simulink model "prius_rulebased"  (Simulink 9.0)
settings: Solver=ode4  StartTime=0.0  StopTime=time_final  FixedStep=time_step  RelTol=1e-3  AbsTol=1e-6
values from neighbouring files (symbols this model uses):
  A_frontal = 2.52    [prius_sim_data.m]
  C_d = 0.3    [prius_sim_data.m]
  enable_stop = 1    [prius_sim_data.m]
  eng_consum_fuel = [0 0.654 0.328 0.238 0.232 0.257 0.29 0.323 0.353 0.381 0.407 0.435 0.465 0.501 0.545 0.599 0.665 0.746 0.842 0.957 ... (first row only)    [prius_sim_data.m]
  eng_ctrl_max_trq = [77.33 78.2 79.07 79.94 80.81 81.68 82.35 82.85 83.35 83.85              84.35 84.83 85.2 85.58 85.95 86.32 86.7 87.13 87.6 88.08 88.55              89.02 89.47 89.79 90.11 90.43 90.76 91.08 91.4 91.73 92.05 92.38              92.7 93.03 93.35 93.67 93.99 94.32 94.64 94.96 95.29 95.61 95.93              96.26 96.58 96.9 97.22 97.55 97.87 98.19 98.52 98.84 99.17 99.49              99.81 100.2 100.5 ...(+23 chars)    [prius_sim_init.m]
  eng_idle_spd = 1000*pi/30    (= 104.71975512)    [prius_sim_init.m]
  eng_pwr_max = 40000    [prius_sim_init.m]
  eng_pwr_opt = eng_spd_opt.*eng_ctrl_max_trq*0.9    [prius_sim_init.m]
  eng_spd_opt = eng_ctrl_spd    [prius_sim_init.m]
  ess_cap_scale = 1    [prius_sim_data.m]
  ess_fixtemp = 40    [prius_sim_data.m]
  ess_init_soc = soc_init_index(simrun)    [prius_sim_init.m]
  ess_max_ah_cap = [6.0 6.0]    [prius_sim_data.m]
  ess_max_volts = 9    [prius_sim_data.m]
  ess_min_volts = 6    [prius_sim_data.m]
  ess_module_num = 40    [prius_sim_data.m]
  ess_res_scale_coef = [1 0 1 0]    [prius_sim_data.m]
  ess_res_scale_fun = inline('(x(1)*ess_module_num+x(2))/(x(3)*ess_cap_scale+x(4))','x','ess_module_num','ess_cap_scale')    [prius_sim_data.m]
  ess_tmp = [0 25]    [prius_sim_data.m]
  f_rolling = 0.015    [prius_sim_data.m]
  FR = 3.905    [prius_sim_data.m]
  g_eff_map = 0.95*[ 0.88	0.89	0.90	0.91	0.90	0.79	0.79	0.79	0.90	0.91	0.90	0.89	0.88 ... (first row only)    [prius_sim_data.m]
  g_gravity = 9.81    [prius_sim_data.m]
  g_max_spd = [-200000 -10000 -8000 -6500 -5500 -4000 -3500 -3000 -2500 -2000 -1500 -1000 -500 0 500 1000 1500 2000 2500 3000 3500 4000 5500 6500 8000 10000 200000]*(2*pi)/60    [prius_sim_data.m]
  g_max_trq = 1.2*[0.01 14.3 18 22 26 36 41 48 55 55 55 55 55 55 55 55 55 55 55 48 41 36 26 22 18 14.3 0.01]    [prius_sim_data.m]
  gc_ki_on = 0.005    [prius_sim_init.m]
  gc_kp_on = 0.9    [prius_sim_init.m]
  gear_no = 4    [prius_sim_data.m]
  Kp_c = 30    [prius_sim_init.m]
  m_eff_map = 0.95*[ .905    .905    .905    .905    .905    .905    .905    .905    .905    .905    .905    .905	.905    .905    .905    .905    .905    .905    .905    .905    .905    .905    .905 ... (first row only)    [prius_sim_data.m]
  m_map_spd = [0 500 1000 1500 2000 2500 3000 3500 4000 4500  6000]*(2*pi)/60    [prius_sim_data.m]
  m_max_trq = interp1(m_spd_data,m_max_trq_data,m_map_spd,'linear')    [prius_sim_data.m]
  m_min_volts = 60    [prius_sim_data.m]
  M_total = 1.254*10^3    (= 1254)    [prius_sim_data.m]
  max_gen_spd = 6500*pi/30    (= 680.678408278)    [prius_sim_init.m]
  min_gen_spd = -6500*pi/30    (= -680.678408278)    [prius_sim_init.m]
  P_eng_mode = 40000    [prius_sim_init.m]
  P_ev_mode = 12000    [prius_sim_init.m]
  R_tire = 0.287    [prius_sim_data.m]
  regstop_soc = 0.8    [prius_sim_init.m]
  rho_air = 1.2    [prius_sim_data.m]
  soc_control = 0.55    [prius_sim_init.m]
  T2W = inv(W2T)    [prius_sim_data.m]
  target_soc = 0.6    [prius_sim_init.m]
  Ti_c = 60    [prius_sim_init.m]
  time_final = 1*length(cyc_mph(:,2))-1    [prius_sim_init.m]
  Tt_c = 65    [prius_sim_init.m]
  tx_pg_r = 78    [prius_sim_data.m]
  tx_pg_s = 30    [prius_sim_data.m]
  v_max_c = 100    [prius_sim_init.m]
  w_engine_on = 30*1600/3600/R_tire    [prius_sim_init.m]
undefined symbols (not defined in the file or in its folder): eng_map_trq
undefined symbols (not defined in the file): ess_r_chg, ess_r_dis, ess_soc, ess_voc
(part 1 of 2)
settings Model: SuppressorTable=22 serialization::archive 11 0 6 0 0 0 0 0  Creator=Yifan  LastModifiedBy=Yifan  ExtModeTrigMode=oneshot  ExtModeArmWhenConnect=off
settings SolverCC: InitialStep=0.001
settings DataIOCC: SignalLoggingSaveFormat=ModelDataLogs  SaveOutput=off  SaveTime=off  SignalLoggingName=sigsOut
settings OptimizationCC: BooleanDataType=off  OptimizeBlockIOStorage=off  BufferReuse=off  GlobalBufferReuse=off  ExpressionFolding=off  LocalBlockOutputs=off  InitFltsAndDblsToZero=on
settings DebuggingCC: SaveWithParameterizedLinksMsg=none  SignalResolutionControl=TryResolveAllWithWarning  MultiTaskDSMMsg=warning  MultiTaskCondExecSysMsg=none
settings HardwareCC: TargetUnknown=on
settings GRTTargetCC: TargetFcnLib=ansi_tfl_tmw.mat  CombineOutputUpdateFcns=off  GRTInterface=on

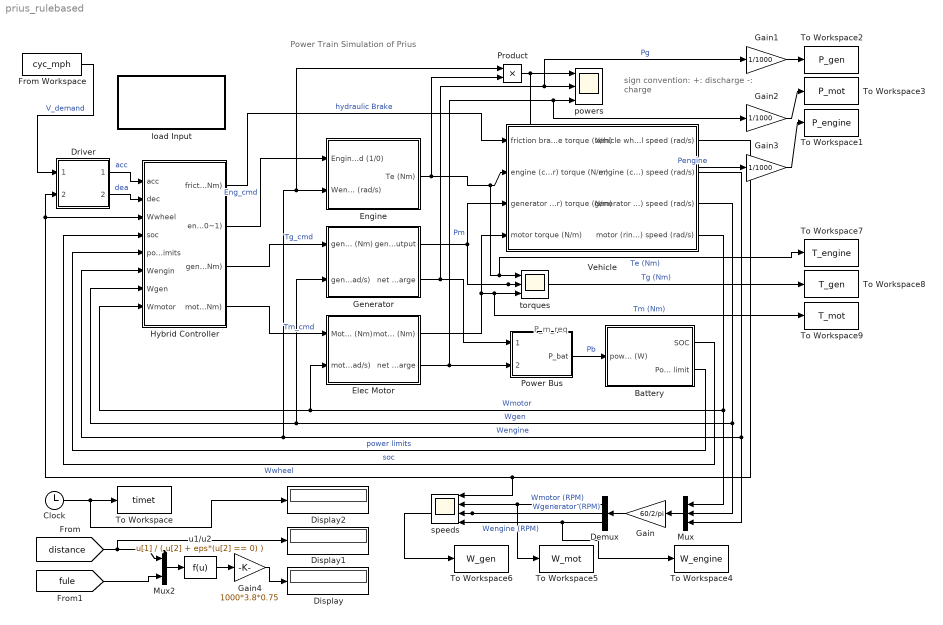
== system prius_rulebased ==
  note: Power Train Simulation of Prius
  note: P_m_req
  note: sign convention:
      | +: discharge     -: charge
  Battery : Subsystem
      mask Display: disp('Battery')
  Clock : Clock
  Demux : Demux  Outputs=3
  Display : Display
  Display1 : Display
  Display2 : Display
  "Driver " : Subsystem
      mask Display: disp('Driver')
  Elec Motor : Subsystem
      mask Display: disp('Electric\nMotor')
  Engine : Subsystem
      mask Display: disp('Engine')
  From Workspace : FromWorkspace  VariableName=cyc_mph  SampleTime=0
  Gain : Gain  Gain=60/2/pi  SaturateOnIntegerOverflow=on  OutDataTypeStr=Inherit: Same as input  ParamDataTypeStr=Inherit: Same as input
  Gain1 : Gain  Gain=1/1000  SaturateOnIntegerOverflow=on  OutDataTypeStr=Inherit: Same as input  ParamDataTypeStr=Inherit: Same as input
  Gain2 : Gain  Gain=1/1000  SaturateOnIntegerOverflow=on  OutDataTypeStr=Inherit: Same as input  ParamDataTypeStr=Inherit: Same as input
  Gain3 : Gain  Gain=1/1000  SaturateOnIntegerOverflow=on  OutDataTypeStr=Inherit: Same as input  ParamDataTypeStr=Inherit: Same as input
  Gain4 : Gain  Gain=1000*3.8*0.75  SaturateOnIntegerOverflow=on  OutDataTypeStr=Inherit: Same as input  ParamDataTypeStr=Inherit: Same as input
  Generator : Subsystem
      mask Display: disp('Generator')
  Hybrid Controller : Subsystem
      mask Display: disp('Hybrid\nController')
  Mux : Mux  Inputs=3
  Mux2 : Mux  Inputs=2
  Power Bus : Subsystem
      mask Display: disp('Power\nBus')
  Product : Product  SaturateOnIntegerOverflow=on  OutDataTypeStr=Inherit: Same as first input
  To Workspace : ToWorkspace  VariableName=timet  SampleTime=-1
  To Workspace1 : ToWorkspace  VariableName=P_engine  SampleTime=-1
  To Workspace2 : ToWorkspace  VariableName=P_gen  SampleTime=-1
  To Workspace3 : ToWorkspace  VariableName=P_mot  SampleTime=-1
  To Workspace4 : ToWorkspace  VariableName=W_engine  SampleTime=-1
  To Workspace5 : ToWorkspace  VariableName=W_mot  SampleTime=-1
  To Workspace6 : ToWorkspace  VariableName=W_gen  SampleTime=-1
  To Workspace7 : ToWorkspace  VariableName=T_engine  SampleTime=-1
  To Workspace8 : ToWorkspace  VariableName=T_gen  SampleTime=-1
  To Workspace9 : ToWorkspace  VariableName=T_mot  SampleTime=-1
  Vehicle : Subsystem
      mask Display: disp('Planetary Gear Set\n&\nVehicle')
  load Input : Subsystem
      settings: OpenFcn=prius_sim_init
      mask Help: This block runs/ndes_init.m file in the main directory
      mask Display: disp('Load Input Data')
  powers : Scope  NumInputPorts=3
  speeds : Scope  NumInputPorts=4
  torques : Scope  NumInputPorts=3
  u1/u2 : Fcn  Expr=u[1] / ( u[2] + eps*(u[2] == 0) )
  wires:
  Power Bus/1(P_bat) -> Battery/1(power req'd into bus (W))  "Pb"
  Battery/1(SOC) -> Hybrid Controller/4(soc)  "soc"
  Hybrid Controller/2(engine command (0~1)) -> Engine/1(Engine on/off cmd (1/0))  "Eng_cmd"
  Hybrid Controller/3(generator torque command (Nm)) -> Generator/1(generator command Torque (Nm))  "Tg_cmd"
  Hybrid Controller/4(motor torque command (Nm)) -> Elec Motor/1(Motor demand Torque (Nm))  "Tm_cmd"
  Elec Motor/2(net Power >0 discharge  <0 charge) -> Power Bus/2(P_motor), powers/3, Gain2/1  "Pm"
  Generator/2(net Power <0 discharge  >0 charge) -> Power Bus/1(P_generator), powers/2, Gain1/1  "Pg"
  Hybrid Controller/1(friction brake torque (Nm)) -> Vehicle/1(friction brake torque (N/m))  "hydraulic Brake"
  Engine/1(Te (Nm)) -> torques/1, To Workspace7/1, Vehicle/2(engine (carrier) torque (N/m)), Product/2  "Te (Nm)"
  Vehicle/1(vehicle wheel speed (rad/s)) -> speeds/1, "Driver "/2(Velocity (rad/s)), Hybrid Controller/3(Wwheel)  "Wwheel"
  Vehicle/2(engine (carrier) speed (rad/s)) -> Hybrid Controller/6(Wengin), Engine/2(Wengine (rad/s)), Product/1, Mux/3  "Wengine"
  Vehicle/3(generator (sun gear) speed (rad/s)) -> Hybrid Controller/7(Wgen), Generator/2(generator speed (rad/s)), Mux/2  "Wgen"
  "Driver "/1(Accel Comd) -> Hybrid Controller/1(acc)  "acc"
  "Driver "/2(Brake Comd) -> Hybrid Controller/2(dec)  "dea"
  Vehicle/4(motor (ring gear) speed (rad/s)) -> Elec Motor/2(motor speed (rad/s)), Hybrid Controller/8(Wmotor), Mux/1  "Wmotor"
  Generator/1(generator torque output) -> torques/2, To Workspace8/1, Vehicle/3(generator (sun gear) torque (N/m))  "Tg (Nm)"
  Elec Motor/1(motor torque output (Nm)) -> torques/3, To Workspace9/1, Vehicle/4(motor torque (N/m))  "Tm (Nm)"
  Battery/2(Power limit) -> Hybrid Controller/5(power limits)  "power limits"
  Product/1 -> powers/1, Gain3/1  "Pengine"
  From Workspace/1 -> "Driver "/1(speed_desired)  "V_demand"
  Gain/1 -> Demux/1
  Mux/1 -> Gain/1
  Demux/1 -> speeds/2, To Workspace5/1  "Wmotor (RPM)"
  Demux/2 -> To Workspace6/1, speeds/3  "Wgenerator (RPM)"
  Demux/3 -> speeds/4, To Workspace4/1  "Wengine (RPM)"
  Clock/1 -> To Workspace/1, Display2/1
  Gain1/1 -> To Workspace2/1
  Gain2/1 -> To Workspace3/1
  Gain3/1 -> To Workspace1/1
  [distance] -> Display1/1, Mux2/1
  [fule] -> Mux2/2
  u1/u2/1 -> Gain4/1
  Gain4/1 -> Display/1
  Mux2/1 -> u1/u2/1

== system prius_rulebased/Battery ==
  note: Assumptions:
      | 1. Constant Temperature
  power req'd into bus (W) : Inport
  Const : Constant  Value=enable_stop
  Mux : Mux  Inputs=2
  Product1 : Product  Inputs=/*  SaturateOnIntegerOverflow=on  InputSameDT=on  OutDataTypeStr=Inherit: Same as first input
  SOC algorithm : Subsystem  AncestorBlock=|
      | lib_energy_storage/Ess Choices/energy
      | storage <ess>/SOC
      | algorithm
      mask Display: disp('SOC\nalgorithm')
  To Workspace : ToWorkspace  VariableName=output_soc  SampleTime=-1
  bat : Scope  NumInputPorts=5
  compute current : Subsystem  AncestorBlock=|
      | lib_energy_storage/Ess Choices/energy
      | storage <ess>/compute
      | current
      mask Display: disp('Compute\nCurrent')
  do ex calcs?1 : Constant  Value=ess_fixtemp
  limit power : Subsystem  AncestorBlock=lib_energy_storage/Ess Choices/energy storage <ess>/limit power
      mask Display: disp('Limit\nPower')
  "pack Voc, Rint" : Subsystem  AncestorBlock=|
      | lib_energy_storage/Ess Choices/energy
      | storage <ess>/pack
      | Voc, Rint
      mask Display: disp('Pack\nVoc,Rint')
  stop sim : Subsystem  AncestorBlock=lib_energy_storage/Ess Choices/energy storage <ess>/stop sim  TreatAsAtomicUnit=on
  SOC : Outport  InitialOutput=0
  Power limit : Outport  Port=2  InitialOutput=0
  wires:
  limit power/1("Pbty, limited") -> compute current/3(limited output power (W))
  "pack Voc, Rint"/1(pack open- circuit voltage) -> limit power/3(Voc), compute current/1(Voc), Product1/1, bat/3  "voc"
  "pack Voc, Rint"/2(pack resistance) -> compute current/2(Rint), limit power/4(Rint)
  Const/1 -> stop sim/Enable
  SOC algorithm/1(SOC1) -> limit power/1(SOC), "pack Voc, Rint"/1(SOC (prev)), SOC/1, To Workspace/1, bat/1, stop sim/1(SOC)  "soc"
  compute current/1(I_) -> SOC algorithm/1((A)), bat/4  "Iout"
  power req'd into bus (W)/1 -> "pack Voc, Rint"/2(req'd battery power (W)), limit power/2(Pbty)
  compute current/2(V_) -> Product1/2
  do ex calcs?1/1 -> "pack Voc, Rint"/3(mod tmp   (C)), SOC algorithm/2(tmp (C))
  Mux/1 -> Power limit/1, bat/5
  Product1/1 -> bat/2  "Power Eff=vout/voc"
  [ess_max_dis_pwr] -> Mux/2
  [ess_max_chg_pwr] -> Mux/1

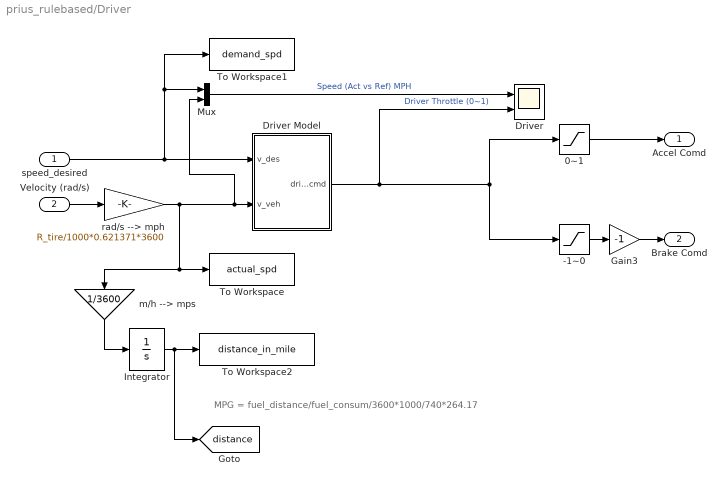
== system prius_rulebased/Driver  ==
  note: MPG = fuel_distance/fuel_consum/3600*1000/740*264.17
  speed_desired : Inport
  Velocity (rad/s) : Inport  Port=2
  -1~0 : Saturate  UpperLimit=0  LowerLimit=-1
  0~1 : Saturate  UpperLimit=1  LowerLimit=0
  Driver : Scope  NumInputPorts=2
  Driver Model : Subsystem
  Gain3 : Gain  Gain=-1  SaturateOnIntegerOverflow=on  OutDataTypeStr=Inherit: Same as input  ParamDataTypeStr=Inherit: Same as input
  Integrator : Integrator  LowerSaturationLimit=0
  Mux : Mux  Inputs=2
  To Workspace : ToWorkspace  VariableName=actual_spd  SampleTime=-1
  To Workspace1 : ToWorkspace  VariableName=demand_spd  SampleTime=-1
  To Workspace2 : ToWorkspace  VariableName=distance_in_mile  SampleTime=time_final
  m/h --> mps : Gain  Gain=1/3600  SaturateOnIntegerOverflow=on  OutDataTypeStr=Inherit: Same as input  ParamDataTypeStr=Inherit: Same as input
  rad/s --> mph : Gain  Gain=R_tire/1000*0.621371*3600  SaturateOnIntegerOverflow=on  OutDataTypeStr=Inherit: Same as input  ParamDataTypeStr=Inherit: Same as input
  Accel Comd : Outport  InitialOutput=0
  Brake Comd : Outport  Port=2  InitialOutput=0
  tag scope: distance=global
  wires:
  speed_desired/1 -> Driver Model/1(v_des), To Workspace1/1, Mux/1
  Velocity (rad/s)/1 -> rad/s --> mph/1
  rad/s --> mph/1 -> To Workspace/1, m/h --> mps/1, Driver Model/2(v_veh), Mux/2
  Driver Model/1(driver_cmd) -> Driver/2, 0~1/1, -1~0/1  "Driver Throttle (0~1)"
  -1~0/1 -> Gain3/1
  0~1/1 -> Accel Comd/1
  Gain3/1 -> Brake Comd/1
  Mux/1 -> Driver/1  "Speed (Act vs Ref) MPH"
  Integrator/1 -> To Workspace2/1, [distance]
  m/h --> mps/1 -> Integrator/1

== system prius_rulebased/Elec Motor ==
  note: disch
  note: charge
  note: discharging
      | power
  Motor demand Torque (Nm) : Inport
  motor speed (rad/s) : Inport  Port=2
  Abs : Abs  SaturateOnIntegerOverflow=on
  Efficiency Look-Up Table (2-D) : Lookup2D  DialogController=Simulink.DDGSource  RowIndex=m_map_spd  ColumnIndex=m_map_trq  Table=m_eff_map  SaturateOnIntegerOverflow=on  InputSameDT=on
  First-order lag : TransferFcn  Denominator=[0.05 1]
  MinMax : MinMax  Inputs=2  SaturateOnIntegerOverflow=on  InputSameDT=on
  Power out  is > 0 or < 0 ? : Switch  SaturateOnIntegerOverflow=on  InputSameDT=on
  Product1 : Product  Inputs=*/  SaturateOnIntegerOverflow=on  InputSameDT=on  OutDataTypeStr=Inherit: Same as first input
  Sign : Signum
  charging power : Product  SaturateOnIntegerOverflow=on  InputSameDT=on  OutDataTypeStr=Inherit: Same as first input
  max torque : Lookup  DialogController=Simulink.DDGSource  InputValues=m_map_spd  Table=m_max_trq  SaturateOnIntegerOverflow=on
  motoring or braking torque2 : Product  SaturateOnIntegerOverflow=on  InputSameDT=on  OutDataTypeStr=Inherit: Same as first input
  power1 : Product  SaturateOnIntegerOverflow=on  InputSameDT=on  OutDataTypeStr=Inherit: Same as first input
  motor torque output (Nm) : Outport  InitialOutput=0
  net Power >0 discharge  <0 charge : Outport  Port=2  InitialOutput=0
  wires:
  charging power/1 -> Power out  is > 0 or < 0 ?/3
  Product1/1 -> Power out  is > 0 or < 0 ?/1
  Power out  is > 0 or < 0 ?/1 -> net Power >0 discharge  <0 charge/1  "power to/from battery (W)"
  motor speed (rad/s)/1 -> Efficiency Look-Up Table (2-D)/1, motoring or braking torque2/1, max torque/1  "motor speed"
  Motor demand Torque (Nm)/1 -> Abs/1, Sign/1
  power1/1 -> First-order lag/1  "torque"
  Efficiency Look-Up Table (2-D)/1 -> Product1/2, charging power/2
  motoring or braking torque2/1 -> Product1/1, charging power/1, Power out  is > 0 or < 0 ?/2
  Abs/1 -> MinMax/2
  max torque/1 -> MinMax/1
  MinMax/1 -> power1/1
  Sign/1 -> power1/2
  First-order lag/1 -> Efficiency Look-Up Table (2-D)/2, motoring or braking torque2/2, motor torque output (Nm)/1

== system prius_rulebased/Engine ==
  note: MPG = fuel_distance/fuel_consum/3600*1000/740*264.17
  Engine on/off cmd (1/0) : Inport
  Wengine (rad/s) : Inport  Port=2
  Integrator : Integrator  UpperSaturationLimit=20.5  LowerSaturationLimit=0
  To Workspace : ToWorkspace  VariableName=fuel_consum_in_g  SampleTime=time_final
  "We, Te to fuel" : Lookup2D  DialogController=Simulink.DDGSource  RowIndex=eng_consum_spd  ColumnIndex=eng_consum_trq  Table=eng_consum_fuel  SaturateOnIntegerOverflow=on  InputSameDT=on
  "fuel, speed to T" : Lookup2D  DialogController=Simulink.DDGSource  RowIndex=eng_map_spd  ColumnIndex=eng_map_fuel  Table=eng_map_trq  SaturateOnIntegerOverflow=on  InputSameDT=on
  Te (Nm) : Outport
  tag scope: fule=global
  wires:
  Engine on/off cmd (1/0)/1 -> "fuel, speed to T"/2
  Wengine (rad/s)/1 -> "fuel, speed to T"/1, "We, Te to fuel"/1
  "fuel, speed to T"/1 -> Te (Nm)/1, "We, Te to fuel"/2
  "We, Te to fuel"/1 -> Integrator/1
  Integrator/1 -> To Workspace/1, [fule]

== system prius_rulebased/Generator ==
  note: disch
  note: charge
  note: discharging
      | power
  generator command Torque (Nm) : Inport
  generator speed (rad/s) : Inport  Port=2
  Abs : Abs  SaturateOnIntegerOverflow=on
  Efficiency Look-Up Table (2-D) : Lookup2D  DialogController=Simulink.DDGSource  RowIndex=g_map_spd  ColumnIndex=g_map_trq  Table=g_eff_map  SaturateOnIntegerOverflow=on  InputSameDT=on
  First-order lag : TransferFcn  Denominator=[0.05 1]
  MinMax : MinMax  Inputs=2  SaturateOnIntegerOverflow=on  InputSameDT=on
  Power out  is > 0 or < 0 ? : Switch  SaturateOnIntegerOverflow=on  InputSameDT=on
  Product1 : Product  Inputs=*/  SaturateOnIntegerOverflow=on  InputSameDT=on  OutDataTypeStr=Inherit: Same as first input
  Sign : Signum
  charging power : Product  SaturateOnIntegerOverflow=on  InputSameDT=on  OutDataTypeStr=Inherit: Same as first input
  max torque : Lookup  DialogController=Simulink.DDGSource  InputValues=g_max_spd  Table=g_max_trq  SaturateOnIntegerOverflow=on
  motoring or braking torque2 : Product  SaturateOnIntegerOverflow=on  InputSameDT=on  OutDataTypeStr=Inherit: Same as first input
  power1 : Product  SaturateOnIntegerOverflow=on  InputSameDT=on  OutDataTypeStr=Inherit: Same as first input
  generator torque output : Outport  InitialOutput=0
  net Power <0 discharge  >0 charge : Outport  Port=2  InitialOutput=0
  wires:
  charging power/1 -> Power out  is > 0 or < 0 ?/3
  Product1/1 -> Power out  is > 0 or < 0 ?/1
  Power out  is > 0 or < 0 ?/1 -> net Power <0 discharge  >0 charge/1  "power to/from battery (W)"
  generator speed (rad/s)/1 -> Efficiency Look-Up Table (2-D)/1, motoring or braking torque2/1, max torque/1  "generator speed"
  generator command Torque (Nm)/1 -> Abs/1, Sign/1
  power1/1 -> First-order lag/1  "torque"
  Efficiency Look-Up Table (2-D)/1 -> Product1/2, charging power/2
  motoring or braking torque2/1 -> Product1/1, charging power/1, Power out  is > 0 or < 0 ?/2
  Abs/1 -> MinMax/2
  max torque/1 -> MinMax/1
  MinMax/1 -> power1/1
  Sign/1 -> power1/2
  First-order lag/1 -> generator torque output/1, Efficiency Look-Up Table (2-D)/2, motoring or braking torque2/2

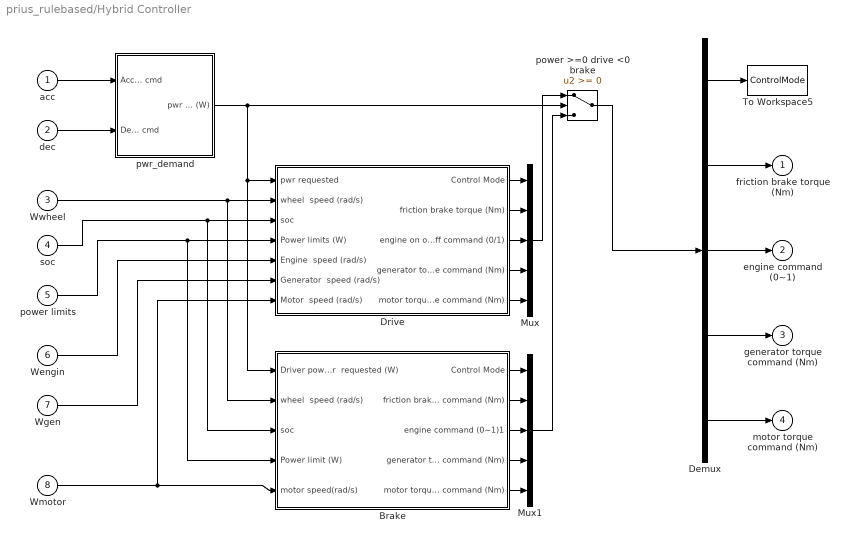
== system prius_rulebased/Hybrid Controller ==
  acc : Inport
  dec : Inport  Port=2
  Wwheel : Inport  Port=3
  soc : Inport  Port=4
  power limits : Inport  Port=5
  Wengin : Inport  Port=6
  Wgen : Inport  Port=7
  Wmotor : Inport  Port=8
  Brake : Subsystem  AncestorBlock=|
      | lib_controls/<vc> prius/Coordinated
      |  Controller/max engine
      | efficiency point
      mask Display: disp('Braking\nControl')
  Demux : Demux  Outputs=5
  Drive : Subsystem  AncestorBlock=|
      | lib_controls/<vc> prius/Coordinated
      |  Controller/max engine
      | efficiency point
      mask Display: disp('Driving\nControl')
  Mux : Mux  Inputs=5
  Mux1 : Mux  Inputs=5
  To Workspace5 : ToWorkspace  VariableName=ControlMode  SampleTime=-1
  power >=0 drive <0 brake : Switch  SaturateOnIntegerOverflow=on
  pwr_demand : Subsystem
      mask Display: disp('Power\nDemand')
  friction brake torque (Nm) : Outport
  engine command (0~1) : Outport  Port=2
  generator torque command (Nm) : Outport  Port=3
  motor torque command (Nm) : Outport  Port=4
  wires:
  pwr_demand/1(pwr dmd (W)) -> Drive/1(pwr requested), Brake/1(Driver power  requested (W)), power >=0 drive <0 brake/2
  acc/1 -> pwr_demand/1(Accel cmd)
  dec/1 -> pwr_demand/2(Decel cmd)
  Drive/1(Control Mode) -> Mux/1
  Drive/2(friction brake torque (Nm)) -> Mux/2
  Drive/3(engine on off command (0/1)) -> Mux/3
  Drive/4(generator torque command (Nm)) -> Mux/4
  Drive/5(motor torque command (Nm)) -> Mux/5
  Brake/1(Control Mode) -> Mux1/1
  Brake/2(friction brake torque command (Nm)) -> Mux1/2
  Brake/3(engine command (0~1)1) -> Mux1/3
  Brake/4(generator torque command (Nm)) -> Mux1/4
  Brake/5(motor torque command (Nm)) -> Mux1/5
  Mux/1 -> power >=0 drive <0 brake/1
  Mux1/1 -> power >=0 drive <0 brake/3
  power >=0 drive <0 brake/1 -> Demux/1
  Demux/1 -> To Workspace5/1
  Demux/2 -> friction brake torque (Nm)/1
  Demux/3 -> engine command (0~1)/1
  Demux/4 -> generator torque command (Nm)/1
  Demux/5 -> motor torque command (Nm)/1
  Wwheel/1 -> Drive/2(wheel  speed (rad/s)), Brake/2(wheel  speed (rad/s))
  soc/1 -> Drive/3(soc), Brake/3(soc)
  power limits/1 -> Drive/4(Power limits (W)), Brake/4(Power limit (W))
  Wengin/1 -> Drive/5(Engine  speed (rad/s))
  Wgen/1 -> Drive/6(Generator  speed (rad/s))
  Wmotor/1 -> Drive/7(Motor  speed (rad/s)), Brake/5(motor speed(rad/s))

== system prius_rulebased/Power Bus ==
  P_generator : Inport
  P_motor : Inport  Port=2
  Gain3 : Gain  Gain=1/1000  SaturateOnIntegerOverflow=on  OutDataTypeStr=Inherit: Same as input  ParamDataTypeStr=Inherit: Same as input
  Sum : Sum  SaturateOnIntegerOverflow=on  InputSameDT=on  OutDataTypeStr=Inherit: Same as first input
  To Workspace : ToWorkspace  VariableName=P_batt  SampleTime=-1
  P_bat : Outport  InitialOutput=0
  wires:
  P_generator/1 -> Sum/1
  P_motor/1 -> Sum/2
  Sum/1 -> P_bat/1, Gain3/1  "Batt"
  Gain3/1 -> To Workspace/1

== system prius_rulebased/Vehicle ==
  friction brake torque (N/m) : Inport
  engine (carrier) torque (N/m) : Inport  Port=2
  generator (sun gear) torque (N/m) : Inport  Port=3
  motor torque (N/m) : Inport  Port=4
  1+tx_pg_r/tx_pg_s : Gain  Gain=1+tx_pg_r/tx_pg_s  SaturateOnIntegerOverflow=on  OutDataTypeStr=Inherit: Same as input  ParamDataTypeStr=Inherit: Same as input
  Dynamics : Subsystem
      mask Display: disp('Dynamic Model\nTwo DOF')
  Sum1 : Sum  Inputs=+-  SaturateOnIntegerOverflow=on  InputSameDT=on  OutDataTypeStr=Inherit: Same as first input
  tx_pg_r/tx_pg_s : Gain  Gain=tx_pg_r/tx_pg_s  SaturateOnIntegerOverflow=on  OutDataTypeStr=Inherit: Same as input  ParamDataTypeStr=Inherit: Same as input
  w_r->w_wh : Fcn  Expr=u/FR
  vehicle wheel speed (rad/s) : Outport
  engine (carrier) speed (rad/s) : Outport  Port=2
  generator (sun gear) speed (rad/s) : Outport  Port=3
  motor (ring gear) speed (rad/s) : Outport  Port=4
  wires:
  tx_pg_r/tx_pg_s/1 -> Sum1/2
  1+tx_pg_r/tx_pg_s/1 -> Sum1/1
  engine (carrier) torque (N/m)/1 -> Dynamics/2(Te: engine (carrier) torque (N/m))
  motor torque (N/m)/1 -> Dynamics/4(Tm: motor torque (N/m))
  friction brake torque (N/m)/1 -> Dynamics/5("Tfb: friction brake torque (N/m) ")
  w_r->w_wh/1 -> vehicle wheel speed (rad/s)/1, Dynamics/1(wheel speed (rad/s))
  generator (sun gear) torque (N/m)/1 -> Dynamics/3(Tg: generator (sun gear) torque (N/m))
  Sum1/1 -> generator (sun gear) speed (rad/s)/1
  Dynamics/1(Carrier speed (rad/s)) -> engine (carrier) speed (rad/s)/1, 1+tx_pg_r/tx_pg_s/1
  Dynamics/2(Ring gear speed (rad/s)) -> w_r->w_wh/1, motor (ring gear) speed (rad/s)/1, tx_pg_r/tx_pg_s/1

== system prius_rulebased/load Input ==
  note: double_click to load

== system prius_rulebased/Battery/SOC algorithm ==
  note: SOC=(Max Ah capacity-Ah used)/Max Ah capacity
  (A) : Inport
  tmp (C) : Inport  Port=2
  (sec->hrs) : Gain  Gain=1/3600  SaturateOnIntegerOverflow=on  OutDataTypeStr=Inherit: Same as input  ParamDataTypeStr=Inherit: Same as input
  0 <= SOC <= 1 : Saturate  UpperLimit=1  LowerLimit=0
  A-h remaining : Sum  Inputs=-+  SaturateOnIntegerOverflow=on  InputSameDT=on  OutDataTypeStr=Inherit: Same as first input
  Ah used : Integrator  InitialConditionSource=external  InitialCondition=(1-ess_init_soc)*ess_max_ah_cap
  Fcn : Fcn  Expr=1/u
  Fcn1 : Fcn  Expr=(1-ess_init_soc)*u
  SOC : Product  SaturateOnIntegerOverflow=on  InputSameDT=on  OutDataTypeStr=Inherit: Same as first input
  max cap : Lookup  DialogController=Simulink.DDGSource  InputValues=ess_tmp  Table=ess_max_ah_cap*ess_cap_scale  SaturateOnIntegerOverflow=on
  SOC1 : Outport  InitialOutput=0
  wires:
  (A)/1 -> (sec->hrs)/1
  (sec->hrs)/1 -> Ah used/1
  Ah used/1 -> A-h remaining/1
  Fcn/1 -> SOC/2
  SOC/1 -> 0 <= SOC <= 1/1
  A-h remaining/1 -> SOC/1
  0 <= SOC <= 1/1 -> SOC1/1
  tmp (C)/1 -> max cap/1
  max cap/1 -> A-h remaining/2, Fcn/1, Fcn1/1
  Fcn1/1 -> Ah used/2

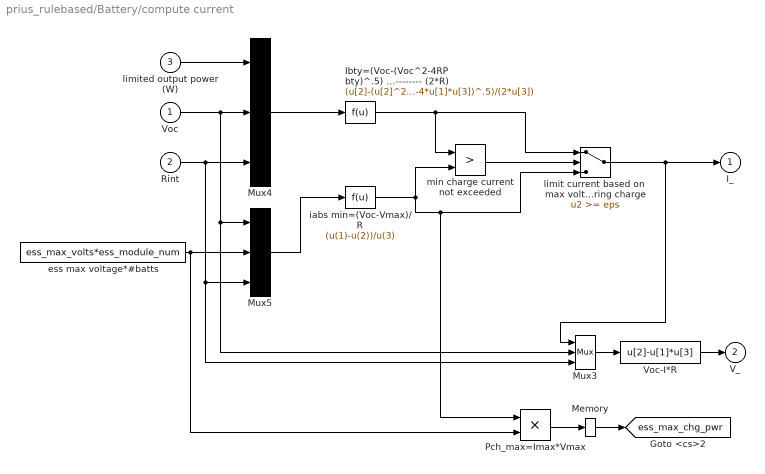
== system prius_rulebased/Battery/compute current ==
  Voc : Inport
  Rint : Inport  Port=2
  limited output power (W) : Inport  Port=3
  Ibty=(Voc-(Voc^2-4RPbty)^.5)        ----------------------------- (2*R) : Fcn  Expr=(u[2]-(u[2]^2-4*u[1]*u[3])^.5)/(2*u[3])
  Memory : Memory
  Mux3 : Mux  Inputs=3
  Mux4 : Mux  Inputs=3
  Mux5 : Mux  Inputs=3
  Pch_max=Imax*Vmax : Product  SaturateOnIntegerOverflow=on  InputSameDT=on  OutDataTypeStr=Inherit: Same as first input
  Voc-I*R : Fcn  Expr=u[2]-u[1]*u[3]
  ess max voltage*#batts : Constant  Value=ess_max_volts*ess_module_num
  iabs min=(Voc-Vmax)/R : Fcn  Expr=(u(1)-u(2))/u(3)
  limit current based on  max voltage during charge : Switch  Threshold=eps  SaturateOnIntegerOverflow=on  InputSameDT=on
  min charge current not exceeded : RelationalOperator  Operator=>  RndMeth=Nearest  InputSameDT=on
  I_ : Outport  InitialOutput=0
  V_ : Outport  Port=2  InitialOutput=0
  tag scope: ess_max_chg_pwr=global
  wires:
  limited output power (W)/1 -> Mux4/1
  Voc/1 -> Mux4/2, Mux3/2, Mux5/1
  Rint/1 -> Mux4/3, Mux3/3, Mux5/3
  Ibty=(Voc-(Voc^2-4RPbty)^.5)        ----------------------------- (2*R)/1 -> min charge current not exceeded/1, limit current based on  max voltage during charge/1
  iabs min=(Voc-Vmax)/R/1 -> min charge current not exceeded/2, limit current based on  max voltage during charge/3, Pch_max=Imax*Vmax/1
  limit current based on  max voltage during charge/1 -> Mux3/1, I_/1
  min charge current not exceeded/1 -> limit current based on  max voltage during charge/2
  Mux3/1 -> Voc-I*R/1
  Voc-I*R/1 -> V_/1
  Mux4/1 -> Ibty=(Voc-(Voc^2-4RPbty)^.5)        ----------------------------- (2*R)/1
  Mux5/1 -> iabs min=(Voc-Vmax)/R/1
  ess max voltage*#batts/1 -> Mux5/2, Pch_max=Imax*Vmax/2
  Pch_max=Imax*Vmax/1 -> Memory/1
  Memory/1 -> [ess_max_chg_pwr]

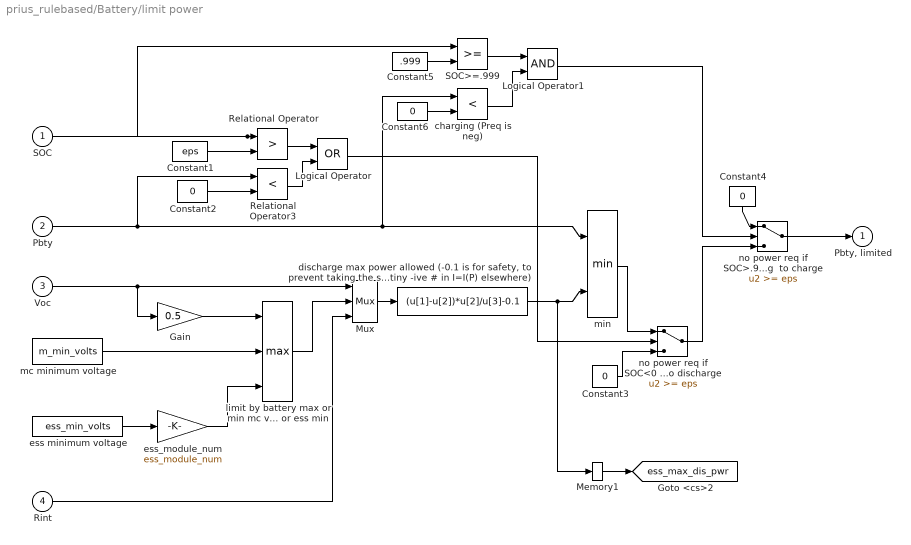
== system prius_rulebased/Battery/limit power ==
  SOC : Inport
  Pbty : Inport  Port=2
  Voc : Inport  Port=3
  Rint : Inport  Port=4
  Constant1 : Constant  Value=eps
  Constant{2..4,6} (4 alike) : Constant  Value=0
  Constant5 : Constant  Value=.999
  Gain : Gain  Gain=0.5  SaturateOnIntegerOverflow=on  OutDataTypeStr=Inherit: Same as input  ParamDataTypeStr=Inherit: Same as input
  Logical Operator : Logic  Operator=OR
  Logical Operator1 : Logic
  Memory1 : Memory
  Mux : Mux  Inputs=3
  Relational Operator : RelationalOperator  Operator=>  RndMeth=Nearest  InputSameDT=on
  Relational Operator3 : RelationalOperator  Operator=<  RndMeth=Nearest  InputSameDT=on
  SOC>=.999 : RelationalOperator  RndMeth=Nearest  InputSameDT=on
  charging (Preq is neg) : RelationalOperator  Operator=<  RndMeth=Nearest  InputSameDT=on
  "discharge max power allowed (-0.1 is for safety, to prevent taking the square of a tiny -ive # in I=I(P) elsewhere)" : Fcn  Expr=(u[1]-u[2])*u[2]/u[3]-0.1
  ess minimum voltage : Constant  Value=ess_min_volts
  ess_module_num : Gain  Gain=ess_module_num  SaturateOnIntegerOverflow=on  OutDataTypeStr=Inherit: Same as input  ParamDataTypeStr=Inherit: Same as input
  limit by battery max or min mc voltage or ess min : MinMax  Function=max  Inputs=3  SaturateOnIntegerOverflow=on  InputSameDT=on
  mc minimum voltage : Constant  Value=m_min_volts
  min : MinMax  Inputs=2  SaturateOnIntegerOverflow=on  InputSameDT=on
  no power req if SOC<0 and trying  to discharge : Switch  Threshold=eps  SaturateOnIntegerOverflow=on  InputSameDT=on
  no power req if SOC>.999 and trying  to charge : Switch  Threshold=eps  SaturateOnIntegerOverflow=on  InputSameDT=on
  "Pbty, limited" : Outport  InitialOutput=0
  tag scope: ess_max_dis_pwr=global
  wires:
  Constant1/1 -> Relational Operator/2
  Relational Operator/1 -> Logical Operator/1
  Pbty/1 -> Relational Operator3/1, charging (Preq is neg)/1, min/1
  Constant2/1 -> Relational Operator3/2
  Relational Operator3/1 -> Logical Operator/2
  Constant3/1 -> no power req if SOC<0 and trying  to discharge/3
  Logical Operator/1 -> no power req if SOC<0 and trying  to discharge/2
  Voc/1 -> Mux/1, Gain/1
  min/1 -> no power req if SOC<0 and trying  to discharge/1
  Mux/1 -> "discharge max power allowed (-0.1 is for safety, to prevent taking the square of a tiny -ive # in I=I(P) elsewhere)"/1
  limit by battery max or min mc voltage or ess min/1 -> Mux/2
  "discharge max power allowed (-0.1 is for safety, to prevent taking the square of a tiny -ive # in I=I(P) elsewhere)"/1 -> min/2, Memory1/1
  mc minimum voltage/1 -> limit by battery max or min mc voltage or ess min/2
  Rint/1 -> Mux/3
  Gain/1 -> limit by battery max or min mc voltage or ess min/1
  ess minimum voltage/1 -> ess_module_num/1
  ess_module_num/1 -> limit by battery max or min mc voltage or ess min/3
  SOC/1 -> Relational Operator/1, SOC>=.999/1
  SOC>=.999/1 -> Logical Operator1/1
  Constant6/1 -> charging (Preq is neg)/2
  charging (Preq is neg)/1 -> Logical Operator1/2
  Constant5/1 -> SOC>=.999/2
  Constant4/1 -> no power req if SOC>.999 and trying  to charge/1
  no power req if SOC<0 and trying  to discharge/1 -> no power req if SOC>.999 and trying  to charge/3
  no power req if SOC>.999 and trying  to charge/1 -> "Pbty, limited"/1
  Logical Operator1/1 -> no power req if SOC>.999 and trying  to charge/2
  Memory1/1 -> [ess_max_dis_pwr]

== system prius_rulebased/Battery/pack Voc, Rint ==
  SOC (prev) : Inport
  req'd battery power (W) : Inport  Port=2
  mod tmp   (C) : Inport  Port=3
  #bty : Constant  Value=ess_module_num
  Product : Product  SaturateOnIntegerOverflow=on  InputSameDT=on  OutDataTypeStr=Inherit: Same as first input
  Rchg (ohms) : Subsystem  mask(2-D Table Lookup){xindex=ess_tmp, yindex=ess_soc, table=ess_r_chg}
      mask prompts: xindex "X Index"; yindex "Y Index"
      mask help:
      | Two Dimensional Table Lookup
      | The first input corresponds to X Index and the second input corresponds to the Y Index
      mask init:
      | sftab2chk(xindex,yindex,table);
      mask Help: This block returns a linearly interpolated intersection from the table using the X index (which corresponds to the rows of the table) and the Y index (which corresponds to the columns of the table).  Extrapolation is used.
      mask Display: plot(-10,-10,110,110,[90,50,10],[90,40,30],[90,50,10],[50,26,20],[90,50,10],[22,13,10])
  Rdis (ohms) : Subsystem  mask(2-D Table Lookup){xindex=ess_tmp, yindex=ess_soc, table=ess_r_dis}
      mask prompts: xindex "X Index"; yindex "Y Index"
      mask help:
      | Two Dimensional Table Lookup
      | The first input corresponds to X Index and the second input corresponds to the Y Index
      mask init:
      | sftab2chk(xindex,yindex,table);
      mask Help: This block returns a linearly interpolated intersection from the table using the X index (which corresponds to the rows of the table) and the Y index (which corresponds to the columns of the table).  Extrapolation is used.
      mask Display: plot(-10,-10,110,110,[90,50,10],[90,40,30],[90,50,10],[50,26,20],[90,50,10],[22,13,10])
  Switch : Switch  SaturateOnIntegerOverflow=on  InputSameDT=on
  VOC (V) : Subsystem  mask(2-D Table Lookup){xindex=ess_tmp, yindex=ess_soc, table=ess_voc}
      mask prompts: xindex "X Index"; yindex "Y Index"
      mask help:
      | Two Dimensional Table Lookup
      | The first input corresponds to X Index and the second input corresponds to the Y Index
      mask init:
      | sftab2chk(xindex,yindex,table);
      mask Help: This block returns a linearly interpolated intersection from the table using the X index (which corresponds to the rows of the table) and the Y index (which corresponds to the columns of the table).  Extrapolation is used.
      mask Display: plot(-10,-10,110,110,[90,50,10],[90,40,30],[90,50,10],[50,26,20],[90,50,10],[22,13,10])
  resistance scale fun : Gain  Gain=ess_res_scale_fun(ess_res_scale_coef,ess_module_num,ess_cap_scale)  SaturateOnIntegerOverflow=on  OutDataTypeStr=Inherit: Same as input  ParamDataTypeStr=Inherit: Same as input
  resistance scale fun1 : Gain  Gain=ess_res_scale_fun(ess_res_scale_coef,ess_module_num,ess_cap_scale)  SaturateOnIntegerOverflow=on  OutDataTypeStr=Inherit: Same as input  ParamDataTypeStr=Inherit: Same as input
  pack open- circuit voltage : Outport  InitialOutput=0
  pack resistance : Outport  Port=2  InitialOutput=0
  wires:
  resistance scale fun1/1 -> Switch/3
  Rchg (ohms)/1(table out) -> resistance scale fun1/1
  resistance scale fun/1 -> Switch/1
  Rdis (ohms)/1(table out) -> resistance scale fun/1
  Switch/1 -> pack resistance/1
  #bty/1 -> Product/2
  Product/1 -> pack open- circuit voltage/1
  VOC (V)/1(table out) -> Product/1
  req'd battery power (W)/1 -> Switch/2
  SOC (prev)/1 -> VOC (V)/2(y0), Rdis (ohms)/2(y0), Rchg (ohms)/2(y0)
  mod tmp   (C)/1 -> VOC (V)/1(x0), Rdis (ohms)/1(x0), Rchg (ohms)/1(x0)

== system prius_rulebased/Battery/stop sim ==
  SOC : Inport
  Enable : EnablePort
  Const : Constant  Value=.001
  Relational Operator : RelationalOperator  Operator=<  RndMeth=Nearest  InputSameDT=on
  Stop Simulation : Stop
  wires:
  Const/1 -> Relational Operator/2
  SOC/1 -> Relational Operator/1
  Relational Operator/1 -> Stop Simulation/1

== system prius_rulebased/Driver /Driver Model ==
  v_des : Inport
  v_veh : Inport  Port=2
  "-1 to 1 " : Saturate  UpperLimit=1  LowerLimit=-1
  1/Ti_c : Gain  Gain=1/Ti_c  SaturateOnIntegerOverflow=on  OutDataTypeStr=Inherit: Same as input  ParamDataTypeStr=Inherit: Same as input
  1/Tt_c : Gain  Gain=1/Tt_c  SaturateOnIntegerOverflow=on  OutDataTypeStr=Inherit: Same as input  ParamDataTypeStr=Inherit: Same as input
  Integrator1 : Integrator
  Kp_c : Gain  Gain=Kp_c  SaturateOnIntegerOverflow=on  OutDataTypeStr=Inherit: Same as input  ParamDataTypeStr=Inherit: Same as input
  Normalize : Gain  Gain=1/v_max_c  SaturateOnIntegerOverflow=on  OutDataTypeStr=Inherit: Same as input  ParamDataTypeStr=Inherit: Same as input
  Normalize1 : Gain  Gain=1/v_max_c  SaturateOnIntegerOverflow=on  OutDataTypeStr=Inherit: Same as input  ParamDataTypeStr=Inherit: Same as input
  Sum1 : Sum  SaturateOnIntegerOverflow=on  InputSameDT=on  OutDataTypeStr=Inherit: Same as first input
  Sum5 : Sum  Inputs=-+  SaturateOnIntegerOverflow=on  InputSameDT=on  OutDataTypeStr=Inherit: Same as first input
  Sum7 : Sum  Inputs=+-  SaturateOnIntegerOverflow=on  InputSameDT=on  OutDataTypeStr=Inherit: Same as first input
  Sum8 : Sum  SaturateOnIntegerOverflow=on  InputSameDT=on  OutDataTypeStr=Inherit: Same as first input
  driver_cmd : Outport
  wires:
  Normalize/1 -> Sum7/1
  v_veh/1 -> Normalize1/1
  Normalize1/1 -> Sum7/2
  v_des/1 -> Normalize/1
  Sum5/1 -> 1/Tt_c/1
  "-1 to 1 "/1 -> Sum5/2, driver_cmd/1
  Integrator1/1 -> Sum1/2
  1/Ti_c/1 -> Sum8/1
  Sum8/1 -> Integrator1/1
  1/Tt_c/1 -> Sum8/2
  Kp_c/1 -> 1/Ti_c/1, Sum1/1
  Sum1/1 -> "-1 to 1 "/1, Sum5/1
  Sum7/1 -> Kp_c/1

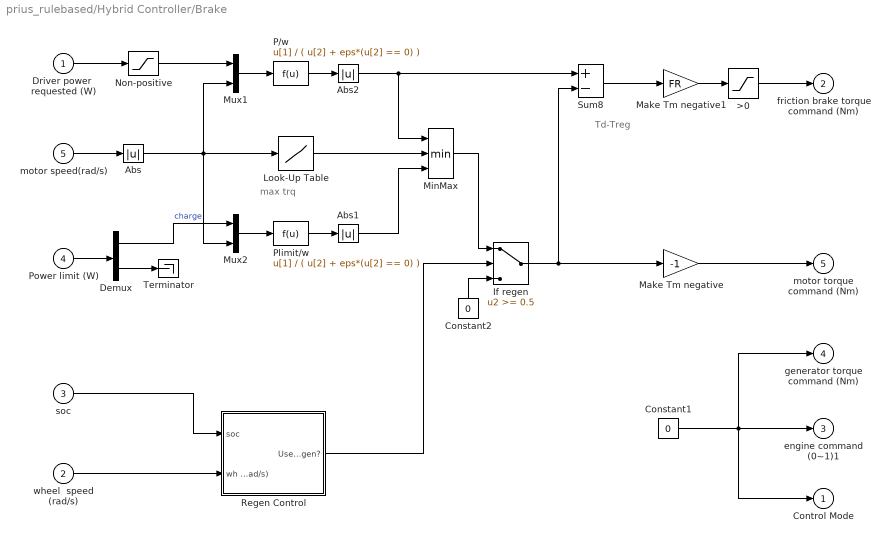
== system prius_rulebased/Hybrid Controller/Brake ==
  note: max trq
  note: Td-Treg
  Driver power  requested (W) : Inport
  wheel  speed (rad/s) : Inport  Port=2
  soc : Inport  Port=3
  Power limit (W) : Inport  Port=4
  motor speed(rad/s) : Inport  Port=5
  >0 : Saturate  UpperLimit=10000  LowerLimit=0
  Abs : Abs  SaturateOnIntegerOverflow=on
  Abs1 : Abs  SaturateOnIntegerOverflow=on
  Abs2 : Abs  SaturateOnIntegerOverflow=on
  Constant1 : Constant  Value=0
  Constant2 : Constant  Value=0
  Demux : Demux  Outputs=2
  If regen : Switch  Threshold=0.5  SaturateOnIntegerOverflow=on  InputSameDT=on
  Look-Up Table : Lookup  DialogController=Simulink.DDGSource  InputValues=m_map_spd  Table=m_max_trq  SaturateOnIntegerOverflow=on
  Make Tm negative : Gain  Gain=-1  SaturateOnIntegerOverflow=on  OutDataTypeStr=Inherit: Same as input  ParamDataTypeStr=Inherit: Same as input
  Make Tm negative1 : Gain  Gain=FR  SaturateOnIntegerOverflow=on  OutDataTypeStr=Inherit: Same as input  ParamDataTypeStr=Inherit: Same as input
  MinMax : MinMax  Inputs=3  SaturateOnIntegerOverflow=on  InputSameDT=on
  Mux1 : Mux  Inputs=2
  Mux2 : Mux  Inputs=2
  Non-positive : Saturate  UpperLimit=0  LowerLimit=-inf
  P/w : Fcn  Expr=u[1] / ( u[2] + eps*(u[2] == 0) )
  Plimit/w : Fcn  Expr=u[1] / ( u[2] + eps*(u[2] == 0) )
  Regen Control : Subsystem
      mask Display: disp('Regen\nControl')
  Sum8 : Sum  Inputs=+-  SaturateOnIntegerOverflow=on  InputSameDT=on  OutDataTypeStr=Inherit: Same as first input
  Terminator : Terminator
  Control Mode : Outport
  friction brake torque command (Nm) : Outport  Port=2
  engine command (0~1)1 : Outport  Port=3
  generator torque command (Nm) : Outport  Port=4
  motor torque command (Nm) : Outport  Port=5
  wires:
  Mux1/1 -> P/w/1
  Non-positive/1 -> Mux1/1
  P/w/1 -> Abs2/1
  Constant2/1 -> If regen/3
  MinMax/1 -> If regen/1
  Demux/1 -> Mux2/1  "charge"
  Power limit (W)/1 -> Demux/1
  If regen/1 -> Make Tm negative/1, Sum8/2
  Abs2/1 -> MinMax/1, Sum8/1
  motor speed(rad/s)/1 -> Abs/1
  Abs/1 -> Look-Up Table/1, Mux1/2, Mux2/2
  Make Tm negative1/1 -> >0/1
  Sum8/1 -> Make Tm negative1/1
  Look-Up Table/1 -> MinMax/2
  wheel  speed (rad/s)/1 -> Regen Control/2(wh spd (rad/s))
  Plimit/w/1 -> Abs1/1
  Abs1/1 -> MinMax/3
  Driver power  requested (W)/1 -> Non-positive/1
  soc/1 -> Regen Control/1(soc)
  >0/1 -> friction brake torque command (Nm)/1
  Make Tm negative/1 -> motor torque command (Nm)/1
  Constant1/1 -> generator torque command (Nm)/1, Control Mode/1, engine command (0~1)1/1
  Mux2/1 -> Plimit/w/1
  Demux/2 -> Terminator/1
  Regen Control/1("Use regen? ") -> If regen/2

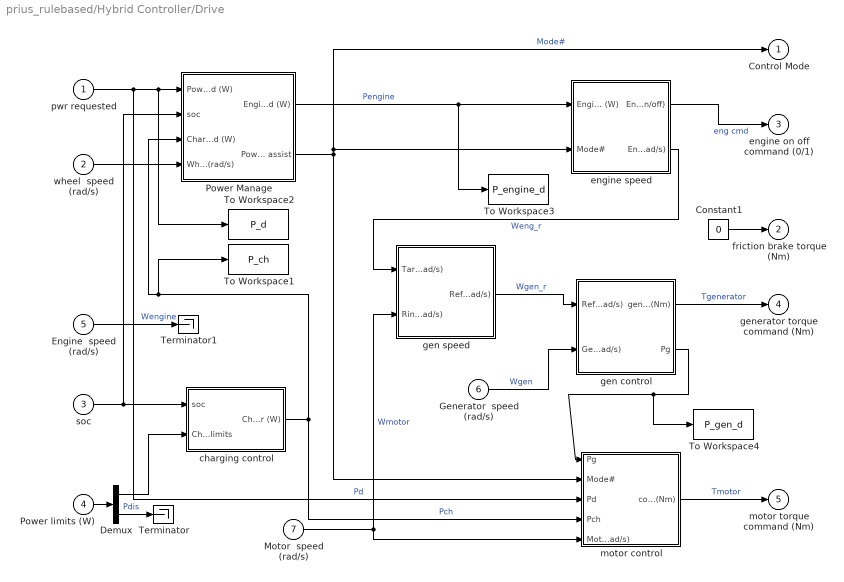
== system prius_rulebased/Hybrid Controller/Drive ==
  pwr requested : Inport
  wheel  speed (rad/s) : Inport  Port=2
  soc : Inport  Port=3
  Power limits (W) : Inport  Port=4
  Engine  speed (rad/s) : Inport  Port=5
  Generator  speed (rad/s) : Inport  Port=6
  Motor  speed (rad/s) : Inport  Port=7
  Constant1 : Constant  Value=0
  Demux : Demux  Outputs=2
  Power Manage : Subsystem
      mask Display: disp('Power\nManagement\nControl')
  Terminator : Terminator
  Terminator1 : Terminator
  To Workspace1 : ToWorkspace  VariableName=P_ch  SampleTime=-1
  To Workspace2 : ToWorkspace  VariableName=P_d  SampleTime=-1
  To Workspace3 : ToWorkspace  VariableName=P_engine_d  SampleTime=-1
  To Workspace4 : ToWorkspace  VariableName=P_gen_d  SampleTime=-1
  charging control : Subsystem  AncestorBlock=|
      | lib_controls/<vc> prius/Coordinated
      |  Controller/max engine
      | efficiency point
      mask Display: disp('Battery\ncharge\nDemand')
  engine speed : Subsystem
      mask Display: disp('Engine\nOptimal\nControl')
  gen control : Subsystem  AncestorBlock=|
      | lib_controls/<vc> prius/Coordinated
      |  Controller/max engine
      | efficiency point
      mask Display: disp('M/G1\nControl')
  gen speed : Subsystem  AncestorBlock=|
      | lib_controls/<vc> prius/Coordinated
      |  Controller/max engine
      | efficiency point
      mask Display: disp('Target\nM/G1\nSpeed')
  motor control : Subsystem  AncestorBlock=|
      | lib_controls/<vc> prius/Coordinated
      |  Controller/max engine
      | efficiency point
      mask Display: disp('M/G2\nControl')
  Control Mode : Outport
  friction brake torque (Nm) : Outport  Port=2
  engine on off command (0/1) : Outport  Port=3
  generator torque command (Nm) : Outport  Port=4
  motor torque command (Nm) : Outport  Port=5
  wires:
  Constant1/1 -> friction brake torque (Nm)/1
  gen control/1(generator torque command (Nm)) -> generator torque command (Nm)/1  "Tgenerator"
  motor control/1(command motor torque (Nm)) -> motor torque command (Nm)/1  "Tmotor"
  gen speed/1(Reference generator speed (rad/s)) -> gen control/1(Reference speed (rad/s))  "Wgen_r"
  Generator  speed (rad/s)/1 -> gen control/2(Generator current  speed (rad/s))  "Wgen"
  soc/1 -> charging control/1(soc), Power Manage/2(soc)
  Power Manage/1(Engine Power demand (W)) -> engine speed/1(Engine Power Demand (W)), To Workspace3/1  "Pengine"
  charging control/1(Charging Power (W)) -> motor control/4(Pch), To Workspace1/1, Power Manage/3(Charging power demand (W))  "Pch"
  Motor  speed (rad/s)/1 -> gen speed/2(Ring Gear/Motor current speed (rad/s)), motor control/5(Motor  speed (rad/s))  "Wmotor"
  pwr requested/1 -> motor control/3(Pd), Power Manage/1(Power demand (W)), To Workspace2/1  "Pd"
  engine speed/1(Engine Cmd (on/off)) -> engine on off command (0/1)/1  "eng cmd"
  engine speed/2(Engine operating speed (rad/s)) -> gen speed/1(Target engine speed (rad/s))  "Weng_r"
  Power Manage/2(Power Mode 1: Motor only 2: Engine only 3: Power assist) -> engine speed/2(Mode#), Control Mode/1, motor control/2(Mode#)  "Mode#"
  Engine  speed (rad/s)/1 -> Terminator1/1  "Wengine"
  Power limits (W)/1 -> Demux/1
  Demux/1 -> charging control/2(Charging power limits)
  wheel  speed (rad/s)/1 -> Power Manage/4(Wheel Speed (rad/s))
  Demux/2 -> Terminator/1  "Pdis"
  gen control/2(Pg) -> To Workspace4/1, motor control/1(Pg)

== system prius_rulebased/Hybrid Controller/pwr_demand ==
  note: max_brake_power
  note: >0:acc; <0:brake
  Accel cmd : Inport
  Decel cmd : Inport  Port=2
  Constant : Constant  Value=55000
  Max braking torqu : Gain  Gain=80000  SaturateOnIntegerOverflow=on  OutDataTypeStr=Inherit: Same as input  ParamDataTypeStr=Inherit: Same as input
  Product : Product  SaturateOnIntegerOverflow=on  InputSameDT=on  OutDataTypeStr=Inherit: Same as first input
  Sum6 : Sum  Inputs=|+-  SaturateOnIntegerOverflow=on  InputSameDT=on  OutDataTypeStr=Inherit: Same as first input
  pwr dmd (W) : Outport
  wires:
  Decel cmd/1 -> Max braking torqu/1
  Accel cmd/1 -> Product/2
  Product/1 -> Sum6/1
  Max braking torqu/1 -> Sum6/2
  Constant/1 -> Product/1  "Max Driving Power (Pengine+Pbattery)"
  Sum6/1 -> pwr dmd (W)/1

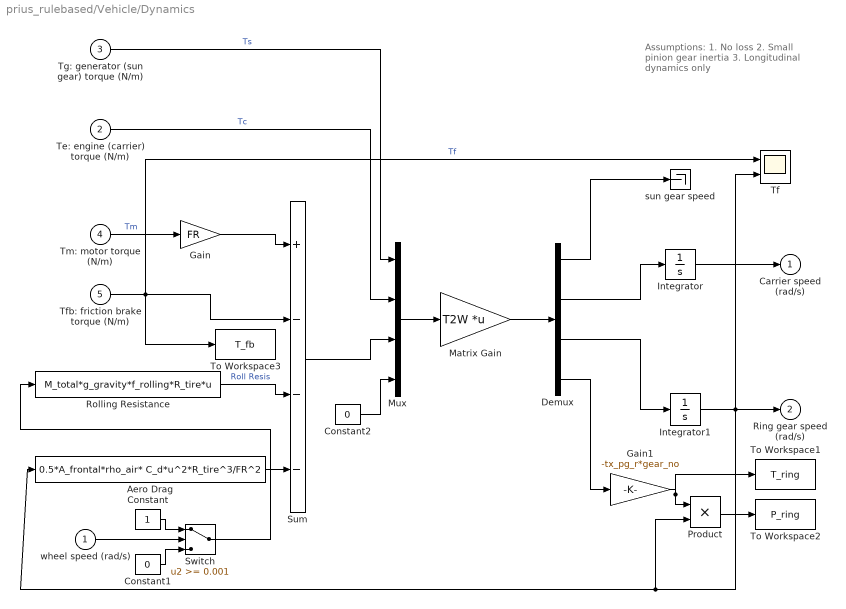
== system prius_rulebased/Vehicle/Dynamics ==
  note: Assumptions:
      | 1. No loss
      | 2. Small pinion gear inertia
      | 3. Longitudinal dynamics only
  wheel speed (rad/s) : Inport
  Te: engine (carrier) torque (N/m) : Inport  Port=2
  Tg: generator (sun gear) torque (N/m) : Inport  Port=3
  Tm: motor torque (N/m) : Inport  Port=4
  "Tfb: friction brake torque (N/m) " : Inport  Port=5
  Aero Drag : Fcn  Expr=0.5*A_frontal*rho_air* C_d*u^2*R_tire^3/FR^2
  Constant : Constant
  Constant1 : Constant  Value=0
  Constant2 : Constant  Value=0
  Demux : Demux
  Gain : Gain  Gain=FR  SaturateOnIntegerOverflow=on  OutDataTypeStr=Inherit: Same as input  ParamDataTypeStr=Inherit: Same as input
  Gain1 : Gain  Gain=-tx_pg_r*gear_no  SaturateOnIntegerOverflow=on  OutDataTypeStr=Inherit: Same as input  ParamDataTypeStr=Inherit: Same as input
  Integrator : Integrator  InitialCondition=1000*2*pi/60  LimitOutput=on  LowerSaturationLimit=0
  Integrator1 : Integrator  LimitOutput=on  LowerSaturationLimit=0
  Matrix Gain : Gain  Gain=T2W  Multiplication=Matrix(K*u)  SaturateOnIntegerOverflow=on  OutDataTypeStr=Inherit: Same as input  ParamDataTypeStr=Inherit: Same as input
  Mux : Mux
  Product : Product  SaturateOnIntegerOverflow=on  InputSameDT=on  OutDataTypeStr=Inherit: Same as first input
  Rolling Resistance : Fcn  Expr=M_total*g_gravity*f_rolling*R_tire*u
  Sum : Sum  Inputs=+---  SaturateOnIntegerOverflow=on
  Switch : Switch  Threshold=0.001  SaturateOnIntegerOverflow=on
  Tf : Scope  NumInputPorts=2
  To Workspace1 : ToWorkspace  VariableName=T_ring  SampleTime=-1
  To Workspace2 : ToWorkspace  VariableName=P_ring  SampleTime=-1
  To Workspace3 : ToWorkspace  VariableName=T_fb  SampleTime=-1
  sun gear speed : Terminator
  Carrier speed (rad/s) : Outport  InitialOutput=0
  Ring gear speed (rad/s) : Outport  Port=2  InitialOutput=0
  wires:
  Demux/2 -> Integrator/1
  Integrator/1 -> Carrier speed (rad/s)/1
  Demux/3 -> Integrator1/1
  Integrator1/1 -> Ring gear speed (rad/s)/1, Tf/2, Aero Drag/1, Product/2
  Rolling Resistance/1 -> Sum/3  "Roll Resis"
  Aero Drag/1 -> Sum/4
  wheel speed (rad/s)/1 -> Switch/2
  Tm: motor torque (N/m)/1 -> Gain/1  "Tm"
  Constant1/1 -> Switch/3
  Constant/1 -> Switch/1
  Switch/1 -> Rolling Resistance/1
  Gain/1 -> Sum/1
  "Tfb: friction brake torque (N/m) "/1 -> Sum/2, Tf/1, To Workspace3/1  "Tf"
  Mux/1 -> Matrix Gain/1
  Tg: generator (sun gear) torque (N/m)/1 -> Mux/1  "Ts"
  Te: engine (carrier) torque (N/m)/1 -> Mux/2  "Tc"
  Sum/1 -> Mux/3
  Constant2/1 -> Mux/4
  Matrix Gain/1 -> Demux/1
  Demux/1 -> sun gear speed/1
  Demux/4 -> Gain1/1
  Gain1/1 -> To Workspace1/1, Product/1
  Product/1 -> To Workspace2/1

== system prius_rulebased/Battery/pack Voc, Rint/Rchg (ohms) ==
  x0 : Inport
  y0 : Inport  Port=2
  Mux : Mux  Inputs=2
  S-function : S-Function  FunctionName=sftable2  Parameters=xindex, yindex, table  SFunctionDeploymentMode=off  EnableBusSupport=off
  table out : Outport  InitialOutput=0
  wires:
  y0/1 -> Mux/2
  S-function/1 -> table out/1
  x0/1 -> Mux/1
  Mux/1 -> S-function/1

== system prius_rulebased/Battery/pack Voc, Rint/Rdis (ohms) ==
  x0 : Inport
  y0 : Inport  Port=2
  Mux : Mux  Inputs=2
  S-function : S-Function  FunctionName=sftable2  Parameters=xindex, yindex, table  SFunctionDeploymentMode=off  EnableBusSupport=off
  table out : Outport  InitialOutput=0
  wires:
  y0/1 -> Mux/2
  S-function/1 -> table out/1
  x0/1 -> Mux/1
  Mux/1 -> S-function/1

== system prius_rulebased/Battery/pack Voc, Rint/VOC (V) ==
  x0 : Inport
  y0 : Inport  Port=2
  Mux : Mux  Inputs=2
  S-function : S-Function  FunctionName=sftable2  Parameters=xindex, yindex, table  SFunctionDeploymentMode=off  EnableBusSupport=off
  table out : Outport  InitialOutput=0
  wires:
  y0/1 -> Mux/2
  S-function/1 -> table out/1
  x0/1 -> Mux/1
  Mux/1 -> S-function/1

== system prius_rulebased/Hybrid Controller/Brake/Regen Control ==
  soc : Inport
  wh spd (rad/s) : Inport  Port=2
  Logical Operator : Logic  Inputs=3
  regen swith on : Constant
  soc condition : Relay  OnSwitchValue=regstop_soc  OffSwitchValue=regstop_soc  OnOutputValue=0  OffOutputValue=1
  wheel spd>= 0.4 : Relay  OnSwitchValue=0.4  OffSwitchValue=0.4
  "Use regen? " : Outport
  wires:
  wh spd (rad/s)/1 -> wheel spd>= 0.4/1
  soc/1 -> soc condition/1
  wheel spd>= 0.4/1 -> Logical Operator/1
  Logical Operator/1 -> "Use regen? "/1
  soc condition/1 -> Logical Operator/2
  regen swith on/1 -> Logical Operator/3

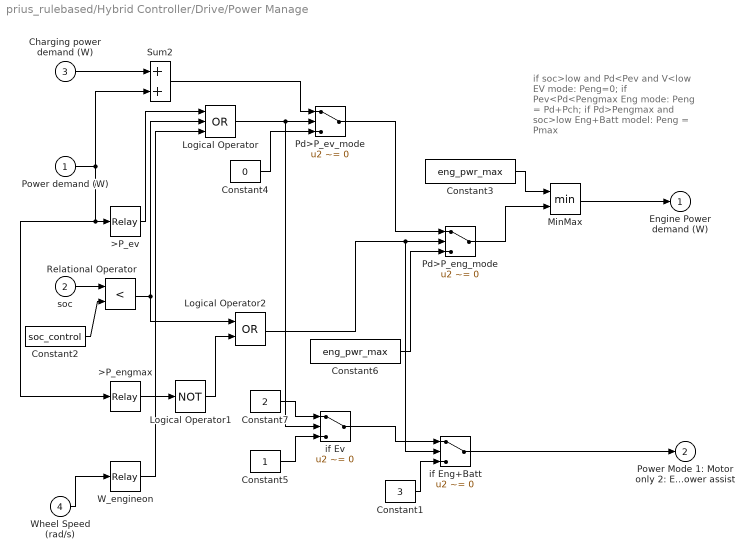
== system prius_rulebased/Hybrid Controller/Drive/Power Manage ==
  note: if soc>low and Pd<Pev and V<low
      |    EV mode:  Peng=0;
      | if Pev<Pd<Pengmax
      |    Eng mode:  Peng = Pd+Pch;
      | if Pd>Pengmax and soc>low
      |    Eng+Batt model:  Peng = Pmax
  Power demand (W) : Inport
  soc : Inport  Port=2
  Charging power demand (W) : Inport  Port=3
  Wheel Speed (rad/s) : Inport  Port=4
  >P_engmax : Relay  OnSwitchValue=P_eng_mode  OffSwitchValue=P_eng_mode*0.9
  >P_ev : Relay  OnSwitchValue=P_ev_mode  OffSwitchValue=P_ev_mode*0.9
  Constant1 : Constant  Value=3
  Constant2 : Constant  Value=soc_control
  Constant3 : Constant  Value=eng_pwr_max
  Constant4 : Constant  Value=0
  Constant5 : Constant
  Constant6 : Constant  Value=eng_pwr_max
  Constant7 : Constant  Value=2
  Logical Operator : Logic  Operator=OR  Inputs=3  AllPortsSameDT=off
  Logical Operator1 : Logic  Operator=NOT  Inputs=3  AllPortsSameDT=off
  Logical Operator2 : Logic  Operator=OR  AllPortsSameDT=off
  MinMax : MinMax  Inputs=2  SaturateOnIntegerOverflow=on  InputSameDT=on
  Pd>P_eng_mode : Switch  Criteria=u2 ~= 0  Threshold=0.5  SaturateOnIntegerOverflow=on  InputSameDT=on
  Pd>P_ev_mode : Switch  Criteria=u2 ~= 0  Threshold=0.5  SaturateOnIntegerOverflow=on  InputSameDT=on
  Relational Operator : RelationalOperator  Operator=<  RndMeth=Nearest
  Sum2 : Sum  SaturateOnIntegerOverflow=on  InputSameDT=on  OutDataTypeStr=Inherit: Same as first input
  W_engineon : Relay  OnSwitchValue=w_engine_on  OffSwitchValue=w_engine_on
  if Eng+Batt : Switch  Criteria=u2 ~= 0  Threshold=0.5  SaturateOnIntegerOverflow=on  InputSameDT=on
  if Ev : Switch  Criteria=u2 ~= 0  Threshold=0.5  SaturateOnIntegerOverflow=on  InputSameDT=on
  Engine Power demand (W) : Outport
  Power Mode 1: Motor only 2: Engine only 3: Power assist : Outport  Port=2
  wires:
  Constant1/1 -> if Eng+Batt/3
  soc/1 -> Relational Operator/1
  Wheel Speed (rad/s)/1 -> W_engineon/1
  Constant2/1 -> Relational Operator/2
  Power demand (W)/1 -> Sum2/2, >P_ev/1, >P_engmax/1
  >P_ev/1 -> Logical Operator/1
  Relational Operator/1 -> Logical Operator/2, Logical Operator2/1
  Constant4/1 -> Pd>P_ev_mode/3
  Logical Operator/1 -> Pd>P_ev_mode/2, if Ev/2
  Charging power demand (W)/1 -> Sum2/1
  Sum2/1 -> Pd>P_ev_mode/1
  >P_engmax/1 -> Logical Operator1/1
  Logical Operator1/1 -> Logical Operator2/2
  Constant6/1 -> Pd>P_eng_mode/3
  Logical Operator2/1 -> Pd>P_eng_mode/2, if Eng+Batt/2
  Pd>P_ev_mode/1 -> Pd>P_eng_mode/1
  Constant3/1 -> MinMax/1
  Pd>P_eng_mode/1 -> MinMax/2
  MinMax/1 -> Engine Power demand (W)/1
  if Eng+Batt/1 -> Power Mode 1: Motor only 2: Engine only 3: Power assist/1
  Constant7/1 -> if Ev/1
  Constant5/1 -> if Ev/3
  if Ev/1 -> if Eng+Batt/1
  W_engineon/1 -> Logical Operator/3
